simulink model "CubeSatModel_nopert"  (R2024a)
settings: Solver=FixedStepAuto  StartTime=0.0  StopTime=5467.6512  FixedStep=0.5  RelTol=1e-6  AbsTol=1e-7
PostLoadFcn:
  | if builtin('license','test','Virtual_Reality_Toolbox')
  |     set_param([bdroot(gcs) '/Simulink 3D Animation'], 'enableVis', 'on')
  | else
  |     set_param([bdroot(gcs) '/Simulink 3D Animation'], 'enableVis', 'off')
  | end
InitFcn:
  | if strcmp(get_param([bdroot(gcs) '/Simulink 3D Animation'], 'enableVis'), 'on')
  |     if ~builtin('license','checkout','Virtual_Reality_Toolbox')
  |         error(message('aeroblks_cubesat:cubesat:licenseFailAnimTemplate'));
  |     end
  | end
model workspace (MATLAB code in the model file + MAT data in the model file):
  aeroCoeff.Cl0 = 0.000591
  aeroCoeff.Cl_beta = -0.0618
  aeroCoeff.Cl_da = -0.09917
  aeroCoeff.Cl_da_alpha = -0.08269
  aeroCoeff.Cl_dr = 0.006934
  aeroCoeff.Cl_p = -0.5045
  aeroCoeff.Cl_r = 0.1695
  aeroCoeff.Cm0 = 0.09448
  aeroCoeff.Cm_alpha = -0.6028
  aeroCoeff.Cm_alpha2 = -2.14
  aeroCoeff.Cm_beta2 = 0.6921
  aeroCoeff.Cm_de = -1.921
  aeroCoeff.Cm_df = 0.4072
  aeroCoeff.Cm_q = -15.56
  aeroCoeff.Cm_r = -0.3118
  aeroCoeff.Cn0 = -0.003117
  aeroCoeff.Cn_beta = 0.006719
  aeroCoeff.Cn_beta3 = 0.1373
  aeroCoeff.Cn_da = -0.003872
  aeroCoeff.Cn_dr = -0.08265
  aeroCoeff.Cn_p = -0.1585
  aeroCoeff.Cn_q = 0.1595
  aeroCoeff.Cn_r = -0.1112
  aeroCoeff.Cx0 = -0.03554
  aeroCoeff.Cx_alpha = 0.00292
  aeroCoeff.Cx_alpha2 = 5.459
  aeroCoeff.Cx_alpha3 = -5.162
  aeroCoeff.Cx_df = -0.09447
  aeroCoeff.Cx_df_alpha = 1.106
  aeroCoeff.Cx_dr = 0.03412
  aeroCoeff.Cx_q = -0.6748
  aeroCoeff.Cy0 = -0.002226
  aeroCoeff.Cy_beta = -0.7678
  aeroCoeff.Cy_da = -0.02956
  aeroCoeff.Cy_dr = 0.1158
  aeroCoeff.Cy_dr_alpha = 0.5238
  aeroCoeff.Cy_p = -0.124
  aeroCoeff.Cy_r = 0.3666
  aeroCoeff.Cz0 = -0.05504
  aeroCoeff.Cz_alpha = -5.578
  aeroCoeff.Cz_alpha3 = 3.442
  aeroCoeff.Cz_de = -0.398
  aeroCoeff.Cz_de_beta = -15.93
  aeroCoeff.Cz_df = -1.377
  aeroCoeff.Cz_df_alpha = -1.261
  aeroCoeff.Cz_q = -2.988
  environment.EarthRefAlt = 0
  initCond.x0 = [0 0 -2202]
  initCond.v0 = [44.54 2.714 5.836]
  initCond.euler0 = [0 0.1308996939 0]
  initCond.w0 = [0 0 0]
  inputs0.time = 0
  inputs0.signals(1).dimensions = 1
  inputs0.signals(1).values = -0.104711430294
  inputs0.signals(2).dimensions = 1
  inputs0.signals(2).values = -0.0698725229544
  inputs0.signals(3).dimensions = 1
  inputs0.signals(3).values = -0.000215042330254
  states0.time = 0
  states0.signals(1).values = [0 0 -2202]
  states0.signals(1).dimensions = 3
  states0.signals(1).label = 'CSTATE'
  states0.signals(1).blockName = 'asb6DOFAirframeTemplate/6DOF EOM/6DOF (Euler Angles)/xe,ye,ze'
  states0.signals(1).stateName = ''
  states0.signals(1).inReferencedModel = 0
  states0.signals(1).sampleTime = [0 0]
  states0.signals(2).values = [0.128665353089 0.259337659946 -0.178947917154]
  states0.signals(2).dimensions = 3
  states0.signals(2).label = 'CSTATE'
  states0.signals(2).blockName = 'asb6DOFAirframeTemplate/6DOF EOM/6DOF (Euler Angles)/Calculate DCM &
    | Euler Angles/phi
    | theta
    | psi'
  states0.signals(2).stateName = ''
  states0.signals(2).inReferencedModel = 0
  states0.signals(2).sampleTime = [0 0]
  states0.signals(3).values = [36.9119692666 8.10720863264 8.82591882596]
  states0.signals(3).dimensions = 3
  states0.signals(3).label = 'CSTATE'
  states0.signals(3).blockName = 'asb6DOFAirframeTemplate/6DOF EOM/6DOF (Euler Angles)/ub,vb,wb'
  states0.signals(3).stateName = ''
  states0.signals(3).inReferencedModel = 0
  states0.signals(3).sampleTime = [0 0]
  states0.signals(4).values = [0 0 0]
  states0.signals(4).dimensions = 3
  states0.signals(4).label = 'CSTATE'
  states0.signals(4).blockName = 'asb6DOFAirframeTemplate/6DOF EOM/6DOF (Euler Angles)/p,q,r '
  states0.signals(4).stateName = ''
  states0.signals(4).inReferencedModel = 0
  states0.signals(4).sampleTime = [0 0]
  states0.signals(5).values = [0 0]
  states0.signals(5).dimensions = 2
  states0.signals(5).label = 'CSTATE'
  states0.signals(5).blockName = 'asb6DOFAirframeTemplate/Environment Model/Dryden Wind Turbulence Model 
    | (Continuous (+q +r))/Filters on velocities/Hwgw(s)/wg_p1'
  states0.signals(5).stateName = ''
  states0.signals(5).inReferencedModel = 0
  states0.signals(5).sampleTime = [0 0]
  states0.signals(6).values = [0 0]
  states0.signals(6).dimensions = 2
  states0.signals(6).label = 'CSTATE'
  states0.signals(6).blockName = 'asb6DOFAirframeTemplate/Environment Model/Dryden Wind Turbulence Model 
    | (Continuous (+q +r))/Filters on velocities/Hwgw(s)/wg_p2'
  states0.signals(6).stateName = ''
  states0.signals(6).inReferencedModel = 0
  states0.signals(6).sampleTime = [0 0]
  states0.signals(7).values = [0 0]
  states0.signals(7).dimensions = 2
  states0.signals(7).label = 'CSTATE'
  states0.signals(7).blockName = 'asb6DOFAirframeTemplate/Environment Model/Dryden Wind Turbulence Model 
    | (Continuous (+q +r))/Filters on velocities/Hvgw(s)/vg_p1'
  states0.signals(7).stateName = ''
  states0.signals(7).inReferencedModel = 0
  states0.signals(7).sampleTime = [0 0]
  states0.signals(8).values = [0 0]
  states0.signals(8).dimensions = 2
  states0.signals(8).label = 'CSTATE'
  states0.signals(8).blockName = 'asb6DOFAirframeTemplate/Environment Model/Dryden Wind Turbulence Model 
    | (Continuous (+q +r))/Filters on velocities/Hvgw(s)/vgw_p2'
  states0.signals(8).stateName = ''
  states0.signals(8).inReferencedModel = 0
  states0.signals(8).sampleTime = [0 0]
  states0.signals(9).values = [0 0]
  states0.signals(9).dimensions = 2
  states0.signals(9).label = 'CSTATE'
  states0.signals(9).blockName = 'asb6DOFAirframeTemplate/Environment Model/Dryden Wind Turbulence Model 
    | (Continuous (+q +r))/Filters on velocities/Hugw(s)/ug_p'
  states0.signals(9).stateName = ''
  states0.signals(9).inReferencedModel = 0
  states0.signals(9).sampleTime = [0 0]
  states0.signals(10).values = [0 0]
  states0.signals(10).dimensions = 2
  states0.signals(10).label = 'CSTATE'
  states0.signals(10).blockName = 'asb6DOFAirframeTemplate/Environment Model/Dryden Wind Turbulence Model 
    | (Continuous (+q +r))/Filters on angular rates/Hrgw/rgw_p'
  states0.signals(10).stateName = ''
  states0.signals(10).inReferencedModel = 0
  states0.signals(10).sampleTime = [0 0]
  states0.signals(11).values = [0 0]
  states0.signals(11).dimensions = 2
  states0.signals(11).label = 'CSTATE'
  states0.signals(11).blockName = 'asb6DOFAirframeTemplate/Environment Model/Dryden Wind Turbulence Model 
    | (Continuous (+q +r))/Filters on angular rates/Hqgw/qgw_p'
  states0.signals(11).stateName = ''
  states0.signals(11).inReferencedModel = 0
  states0.signals(11).sampleTime = [0 0]
  states0.signals(12).values = [0 0]
  states0.signals(12).dimensions = 2
  states0.signals(12).label = 'CSTATE'
  states0.signals(12).blockName = 'asb6DOFAirframeTemplate/Environment Model/Dryden Wind Turbulence Model 
    | (Continuous (+q +r))/Filters on angular rates/Hpgw/pgw_p'
  states0.signals(12).stateName = ''
  states0.signals(12).inReferencedModel = 0
  states0.signals(12).sampleTime = [0 0]
  vehicle.Sref = 23.23
  vehicle.cbar = 1.5875
  vehicle.bref = 14.63
  vehicle.CG = [0 0 0]
  vehicle.CP = [0 0 0]
  vehicle.inertia = [5788  0  117.6; 0  6928.9  0; -117.6  0  11578.3]
  vehicle.acMass = 2288.231
  vehicle.Thrust = 2300
  vehicle.aileron_max = 0.523598775598
  vehicle.aileron_min = -0.523598775598
  vehicle.elevator_max = 0.523598775598
  vehicle.elevator_min = -0.523598775598
  vehicle.rudder_max = 1.0471975512
  vehicle.rudder_min = -1.0471975512
  other statements: initialize6DOFSkyHogg;
libraries: aerolibutil x12, sharedutil x4, aerolibconvert2 x4, aerolibcubesatveh x1, aerolibobsolete x1, aerolibattitudesys x1, simulink x1, vrlib x1
settings Model: Creator=sandr  LastModifiedBy=sandr
settings SolverCC: AlgebraicLoopSolver=TrustRegion  AutoInsertRateTranBlk=on  InsertRTBMode=Never (minimum delay)  MinimalZcImpactIntegration=on  MaxZcPerStep=1
settings DataIOCC: SignalLogging=off  DSMLogging=off  SaveTime=off
settings OptimizationCC: EnhancedBackFolding=on  StrengthReduction=on  InitFltsAndDblsToZero=on  DifferentSizesBufferReuse=on
settings DebuggingCC: WriteAfterWriteMsg=DisableAll  AlgebraicLoopMsg=none  FcnCallInpInsideContextMsg=warning  UniqueDataStoreMsg=error  RootOutportRequireBusObject=none  StateNameClashWarn=warning  PregeneratedLibrarySubsystemCodeDiagnostic=none  StrictBusMsg=ErrorOnBusTreatedAsVector  SFUnexpectedBacktrackingDiag=warning  SFNoUnconditionalDefaultTransitionDiag=warning  SFExecutionAtInitializationDiag=none  ArithmeticOperatorsInVariantConditions=warning
settings ModelReferenceCC: EnableRefExpFcnMdlSchedulingChecks=on  PropagateSignalLabelsOutOfModel=off
settings SFSimCC: SimUseLocalCustomCode=off
settings RTWCC: RTWUseLocalCustomCode=off  GPUComputeCapability=3.5  DLArmComputeVersion=19.05
settings CodeAppCC: StateflowObjectComments=on

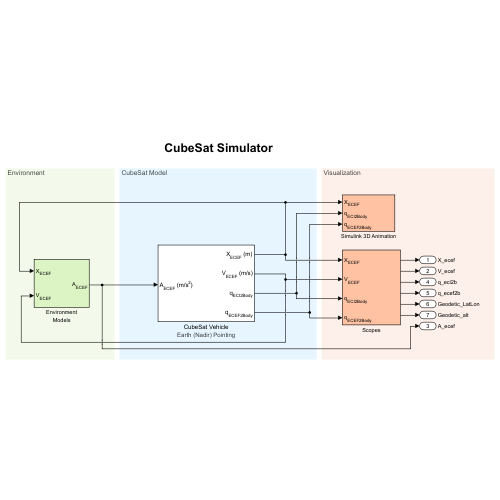
[thumbnail: Simulink's stored preview of the top-level diagram]
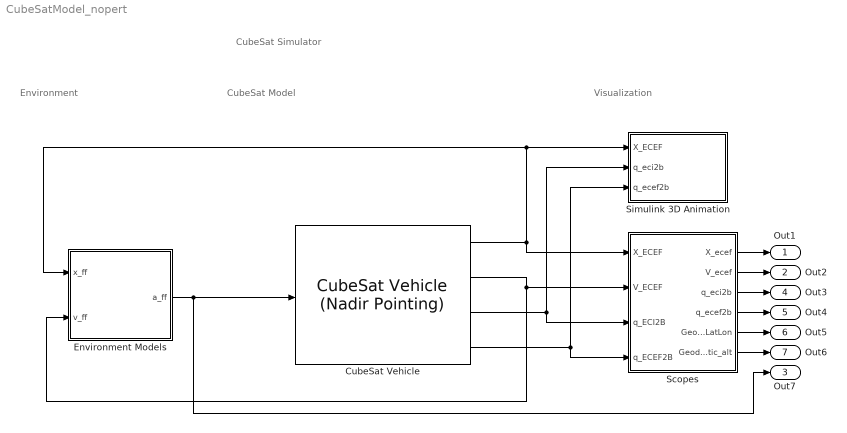
== system CubeSatModel_nopert ==
  note: CubeSat Simulator
  note: Visualization
  note: Environment
  note: CubeSat Model
  CubeSat Vehicle : aerolibcubesatveh/CubeSat Vehicle (Nadir Pointing)  sim_t0=2456824  method=Keplerian Orbital Elements  epoch=2456824  a=mission.CubeSat.SemiMajorAxis  ecc=mission.CubeSat.Eccentricity  incl=mission.CubeSat.Inclination  omega=mission.CubeSat.RAAN  argp=mission.CubeSat.ArgOfPeriapsis  nu=mission.CubeSat.TrueAnomaly  truelon=0  arglat=0  lonper=0  r_eci=[0 0 0]  v_eci=[0 0 0]  r_ecef=[0 0 0]  v_ecef=[0 0 0]  lla=[0 0 0]  v_ned=[0 0 0]  euler=mission.CubeSat.Euler  pqr=mission.CubeSat.AngularRate  pointingMode=Earth (Nadir) Pointing  firstAlignExt=Dialog  firstAlign=[0 0 1]  secondAlignExt=Dialog  secondAlign=[0 1 0]  constraintCoord=ECI Axes  firstRefExt=Dialog  firstRef=[1 0 0]  secondRefExt=Dialog  secondRef=[0 0 1]  missionRTSource=Dialog  missionRT=6*60*60  missionGS=[42, -71]  missionTOICheck=on  missionTOI=[]  missionEta=55
      settings: AttributesFormatString=%<pointingMode>
  Environment Models : Subsystem
      mask Display:
      | port_label('input', 1, 'X_{ECEF}','texmode','on')
      | port_label('input', 2, 'V_{ECEF}','texmode','on')
      | port_label('output', 1, 'A_{ECEF}','texmode','on')
  Scopes : Subsystem  VariantControl=visOff
      mask Display:
      | port_label('input', 1, 'X_{ECEF}','texmode','on')
      | port_label('input', 2, 'V_{ECEF}','texmode','on')
      | port_label('input', 3, 'q_{ECI2Body}','texmode','on')
      | port_label('input', 4, 'q_{ECEF2Body}','texmode','on')
  Simulink 3D Animation : Subsystem  mask(Set Animation Properties){enableVis=on, startDate=2458488, visSampleTime=5, cubesatSize=2e5, showAntenna=on, antennaHeight=1e6, antennaHalfAngle=25}
      mask prompts: enableVis "spacecraft:cubesat:AnimEnableVis"; startDate "spacecraft:cubesat:StartDate"; visSampleTime "spacecraft:cubesat:AnimSampleTime"; cubesatSize "spacecraft:cubesat:MdlSize"; showAntenna "spacecraft:cubesat:ShowCone"; antennaHeight "spacecraft:cubesat:ConeHeight"; antennaHalfAngle "spacecraft:cubesat:ConeAngle"
      mask help: spacecraft:cubesat:VisBlockDesc
      settings: OpenFcn=|
      | if ~builtin('license','test','virtual_reality_toolbox')
      |     set_param(gcb, 'enableVis', 'off');
      | end
      | open_system(gcb,'mask');
      mask Callback enableVis:
      | if strcmp(get_param(gcb,'enableVis'), 'on')
      |     [licAvail, ~] = builtin('license','checkout','Virtual_Reality_Toolbox');
      |     if licAvail
      |         enable = repmat({'on'},7,1);
      |         set_param(gcb, 'Commented', 'off');
      |     else
      |         enable = repmat({'off'},7,1);
      |         set_param(gcb, 'Commented', 'on');
      |         set_param(gcb,'enableVis', 'off');
      |     end
      |     clear licAvail
      | else
      |     enable = repmat({'off'},7,1);
      |     set_param(gcb, 'Commented', 'on');
      | end
      | enable{1} = 'on';
      | set_param(gcb,'MaskEnables', enable);
      | clear enable
      mask Callback showAntenna:
      | if strcmp(get_param(gcb, 'enableVis'), 'on')
      |     enable = get_param(gcb,'MaskEnables');
      |     if strcmp(get_param(gcb, 'showAntenna'), 'off')
      |         enable(6:7) = {'off'};
      |     else
      |         enable(6:7) = {'on'};
      |     end
      |     set_param(gcb,'MaskEnables', enable);
      |     clear enable
      | end
      mask DialogControl enableVis Prompt: Enable visualization with Simulink 3D Animation
      mask DialogControl vrOpenBtn Prompt: spacecraft:cubesat:AnimOpenBtn
      mask DialogControl vrOpenBtn Callback:
      | if builtin('license','checkout','Virtual_Reality_Toolbox')
      |     vrmfunc('FnOpen',getSimulinkBlockHandle([gcb '/VR Sink']));
      | end
      mask DialogControl startDate Prompt: Start date [Julian date]:
      mask DialogControl startDate Tooltip: spacecraft:cubesat:StartDateTT
      mask DialogControl visSampleTime Prompt: Animation refresh rate:
      mask DialogControl visSampleTime Tooltip: spacecraft:cubesat:AnimSampleTimeTT
      mask DialogControl cubesatSize Prompt: CubeSat display size [m]:
      mask DialogControl cubesatSize Tooltip: spacecraft:cubesat:MdlSizeTT
      mask DialogControl Container3 Prompt: spacecraft:cubesat:AntennaPropArea
      mask DialogControl showAntenna Prompt: Show antenna cone in animation
      mask DialogControl showAntenna Tooltip: spacecraft:cubesat:ShowConeTT
      mask DialogControl antennaHeight Prompt: Antenna cone height [m]:
      mask DialogControl antennaHeight Tooltip: spacecraft:cubesat:ConeHeightTT
      mask DialogControl antennaHalfAngle Prompt: Antenna cone half angle [deg]:
      mask DialogControl antennaHalfAngle Tooltip: spacecraft:cubesat:ConeAngleTT
      mask Display:
      | port_label('input', 1, 'X_{ECEF}','texmode','on')
      | port_label('input', 2, 'q_{ECI2Body}','texmode','on')
      | port_label('input', 3, 'q_{ECEF2Body}','texmode','on')
  Out1 : Outport  SignalName=X_ecef
  Out2 : Outport  Port=2  SignalName=V_ecef
  Out7 : Outport  Port=3  SignalName=A_ecef
  Out3 : Outport  Port=4  SignalName=q_eci2b
  Out4 : Outport  Port=5  SignalName=q_ecef2b
  Out5 : Outport  Port=6  SignalName=Geodetic_LatLon
  Out6 : Outport  Port=7  SignalName=Geodetic_alt
  wires:
  Environment Models/1(a_ff) -> Out7/1, CubeSat Vehicle/1
  CubeSat Vehicle/1 -> Scopes/1(X_ECEF), Environment Models/1(x_ff), Simulink 3D Animation/1(X_ECEF)
  CubeSat Vehicle/3 -> Simulink 3D Animation/2(q_eci2b), Scopes/3(q_ECI2B)
  CubeSat Vehicle/2 -> Environment Models/2(v_ff), Scopes/2(V_ECEF)
  CubeSat Vehicle/4 -> Simulink 3D Animation/3(q_ecef2b), Scopes/4(q_ECEF2B)
  Scopes/1(X_ecef) -> Out1/1
  Scopes/2(V_ecef) -> Out2/1
  Scopes/3(q_eci2b) -> Out3/1
  Scopes/4(q_ecef2b) -> Out4/1
  Scopes/5(Geodetic_LatLon) -> Out5/1
  Scopes/6(Geodetic_alt) -> Out6/1

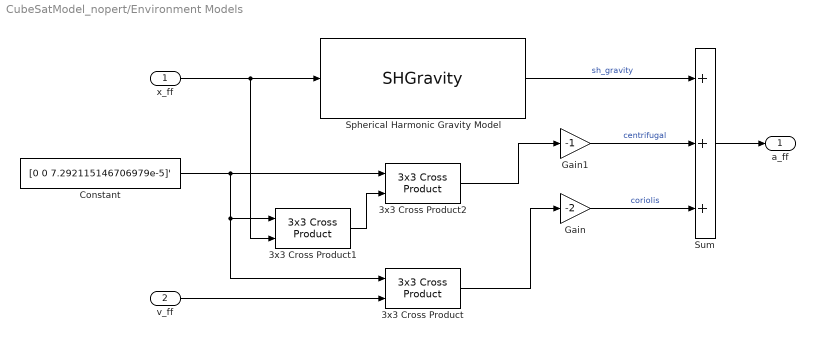
== system CubeSatModel_nopert/Environment Models ==
  x_ff : Inport  Unit=m  PortDimensions=3
  v_ff : Inport  Port=2  Unit=m/s  PortDimensions=3
  3x3 Cross Product : sharedutil/3x3 Cross Product  aMode=aMode
  3x3 Cross Product1 : sharedutil/3x3 Cross Product  aMode=aMode
  3x3 Cross Product2 : sharedutil/3x3 Cross Product  aMode=aMode
  Constant : Constant  Value=[0 0 7.292115146706979e-5]'
  Gain : Gain  Gain=-2
  Gain1 : Gain  Gain=-1
  Spherical Harmonic Gravity Model : SHGravity  degree=40
  Sum : Sum  Inputs=+++
  a_ff : Outport  Unit=m/s^2  PortDimensions=3
  wires:
  Gain/1 -> Sum/3  "coriolis"
  v_ff/1 -> 3x3 Cross Product/2
  x_ff/1 -> Spherical Harmonic Gravity Model/1, 3x3 Cross Product1/2
  Sum/1 -> a_ff/1
  3x3 Cross Product2/1 -> Gain1/1
  Gain1/1 -> Sum/2  "centrifugal"
  Spherical Harmonic Gravity Model/1 -> Sum/1  "sh_gravity"
  3x3 Cross Product1/1 -> 3x3 Cross Product2/2
  Constant/1 -> 3x3 Cross Product2/1, 3x3 Cross Product/1, 3x3 Cross Product1/1
  3x3 Cross Product/1 -> Gain/1

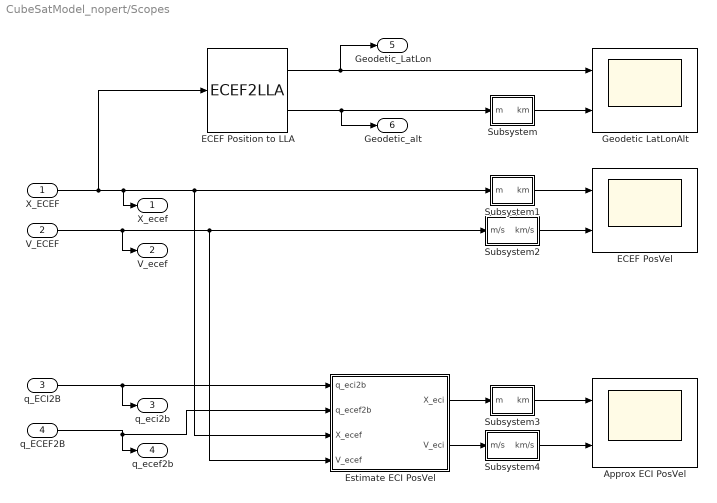
== system CubeSatModel_nopert/Scopes ==
  X_ECEF : Inport
  V_ECEF : Inport  Port=2
  q_ECI2B : Inport  Port=3
  q_ECEF2B : Inport  Port=4
  Approx ECI PosVel : Scope  NumInputPorts=2
  ECEF PosVel : Scope  NumInputPorts=2
  ECEF Position to LLA : ECEF2LLA  R=6378137
  Estimate ECI PosVel : Subsystem
  Geodetic LatLonAlt : Scope  NumInputPorts=2
  Subsystem : Subsystem
  Subsystem1 : Subsystem
  Subsystem2 : Subsystem
  Subsystem3 : Subsystem
  Subsystem4 : Subsystem
  X_ecef : Outport
  V_ecef : Outport  Port=2
  q_eci2b : Outport  Port=3
  q_ecef2b : Outport  Port=4
  Geodetic_LatLon : Outport  Port=5
  Geodetic_alt : Outport  Port=6
  wires:
  V_ECEF/1 -> V_ecef/1, Subsystem2/1(m/s), Estimate ECI PosVel/4(V_ecef)
  X_ECEF/1 -> X_ecef/1, Subsystem1/1(m), Estimate ECI PosVel/3(X_ecef), ECEF Position to LLA/1
  q_ECI2B/1 -> q_eci2b/1, Estimate ECI PosVel/1(q_eci2b)
  Estimate ECI PosVel/2(V_eci) -> Subsystem4/1(m/s)
  Estimate ECI PosVel/1(X_eci) -> Subsystem3/1(m)
  ECEF Position to LLA/2 -> Geodetic_alt/1, Subsystem/1(m)
  Subsystem/1(km) -> Geodetic LatLonAlt/2
  Subsystem1/1(km) -> ECEF PosVel/1
  Subsystem2/1(km/s) -> ECEF PosVel/2
  Subsystem3/1(km) -> Approx ECI PosVel/1
  Subsystem4/1(km/s) -> Approx ECI PosVel/2
  ECEF Position to LLA/1 -> Geodetic LatLonAlt/1, Geodetic_LatLon/1
  q_ECEF2B/1 -> q_ecef2b/1, Estimate ECI PosVel/2(q_ecef2b)

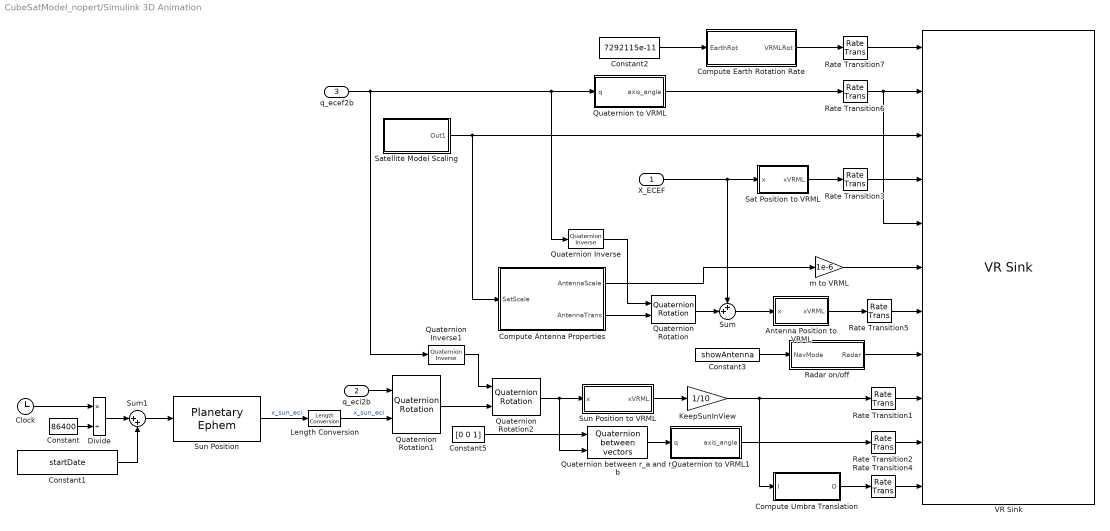
== system CubeSatModel_nopert/Simulink 3D Animation ==
  X_ECEF : Inport
  q_eci2b : Inport  Port=2
  q_ecef2b : Inport  Port=3
  Antenna Position to VRML : Subsystem
  Clock : Clock
  Compute Antenna Properties : Subsystem
  Compute Earth Rotation Rate : Subsystem
  Compute Umbra Translation : Subsystem
  Constant : Constant  Value=86400
  Constant1 : Constant  RequirementInfo={} %GIDa_d3dce1ea_7a4c_4489_9b49_860fce94c68a  Value=startDate  SampleTime=visSampleTime
  Constant2 : Constant  RequirementInfo={} %GIDa_a027479b_4c7b_4f1d_b86b_1fc869131b24  Value=7292115e-11
  Constant3 : Constant  Value=showAntenna
  Constant5 : Constant  Value=[0 0 1]
  Divide : Product  Inputs=*/
  KeepSunInView : Gain  Gain=1/10
  Length Conversion : aerolibconvert2/Length Conversion  IU=km  OU=m
  Quaternion Inverse : aerolibutil/Quaternion Inverse
  Quaternion Inverse1 : aerolibutil/Quaternion Inverse
  Quaternion Rotation : aerolibutil/Quaternion Rotation
  Quaternion Rotation1 : aerolibutil/Quaternion Rotation
  Quaternion Rotation2 : aerolibutil/Quaternion Rotation
  Quaternion between r_a and r_b : aerolibattitudesys/Quaternion between vectors
  Quaternion to VRML : Subsystem
  Quaternion to VRML1 : Subsystem
  Radar on/off : Subsystem
  Rate Transition{1..7} (7 alike) : RateTransition
  Sat Position to VRML : Subsystem
  Satellite Model Scaling : Subsystem
  Sum : Sum  Inputs=++|
  Sum1 : Sum  Inputs=|++
  Sun Position : PlanetaryEphem  ephemerisModel=DE421  target=Sun  outputVelocity=off
  Sun Position to VRML : Subsystem
  VR Sink : vrlib/VR Sink  InstantiateOnLoad=on  SampleTime=visSampleTime  ViewEnable=on  RemoteChange=off  RemoteView=off  FieldsWritten=Earth.rotation.4.1.1.double#Satellite.rotation.4.1.1.double#Satellite.scale.3.1.1.double#Satellite.translation.3.1.1.double#AntennaCone.rotation.4.1.1.double#AntennaCone.scale.3.1.1.double#AntennaCone.translation.3.1.1.double#AntennaMaterial.transparency.1.1.1.double#Sun.translation.3.1.1.double#Umbra.rotation.4.1.1.double#Umbra.translation.3.1.1.double  WorldFileName=cubesatAnim.wrl  WorldDescription=CubeSat Orbit Animation  AutoView=on  VideoDimensions=[]  AllowVariableSize=off
  m to VRML : Gain  Gain=1e-6
  wires:
  Quaternion to VRML1/1(axis_angle) -> Rate Transition2/1
  Quaternion between r_a and r_b/1 -> Quaternion to VRML1/1(q)
  Constant2/1 -> Compute Earth Rotation Rate/1(EarthRot)
  Compute Antenna Properties/1(AntennaScale) -> m to VRML/1
  Quaternion to VRML/1(axis_angle) -> Rate Transition6/1
  Compute Umbra Translation/1(O) -> Rate Transition4/1
  q_eci2b/1 -> Quaternion Rotation1/1
  Quaternion Rotation2/1 -> Sun Position to VRML/1(x), Quaternion between r_a and r_b/2
  Constant5/1 -> Quaternion between r_a and r_b/1
  KeepSunInView/1 -> Compute Umbra Translation/1(I), Rate Transition1/1
  Sun Position to VRML/1(xVRML) -> KeepSunInView/1
  Sat Position to VRML/1(xVRML) -> Rate Transition3/1
  Compute Antenna Properties/2(AntennaTrans) -> Quaternion Rotation/2
  Satellite Model Scaling/1(Out1) -> VR Sink/3, Compute Antenna Properties/1(SatScale)
  Constant3/1 -> Radar on/off/1(NavMode)
  q_ecef2b/1 -> Quaternion Inverse/1, Quaternion to VRML/1(q), Quaternion Inverse1/1
  Quaternion Rotation1/1 -> Quaternion Rotation2/2
  Compute Earth Rotation Rate/1(VRMLRot) -> Rate Transition7/1
  Antenna Position to VRML/1(xVRML) -> Rate Transition5/1
  Quaternion Inverse/1 -> Quaternion Rotation/1
  X_ECEF/1 -> Sat Position to VRML/1(x), Sum/1
  Quaternion Rotation/1 -> Sum/2
  Sum/1 -> Antenna Position to VRML/1(x)
  Quaternion Inverse1/1 -> Quaternion Rotation2/1
  Rate Transition4/1 -> VR Sink/11
  Rate Transition2/1 -> VR Sink/10
  Rate Transition1/1 -> VR Sink/9
  Rate Transition5/1 -> VR Sink/7
  m to VRML/1 -> VR Sink/6
  Rate Transition3/1 -> VR Sink/4
  Rate Transition7/1 -> VR Sink/1
  Rate Transition6/1 -> VR Sink/5, VR Sink/2
  Constant1/1 -> Sum1/2
  Divide/1 -> Sum1/1
  Constant/1 -> Divide/2
  Sun Position/1 -> Length Conversion/1  "x_sun_eci"
  Clock/1 -> Divide/1
  Length Conversion/1 -> Quaternion Rotation1/2  "x_sun_eci"
  Sum1/1 -> Sun Position/1
  Radar on/off/1(Radar) -> VR Sink/8

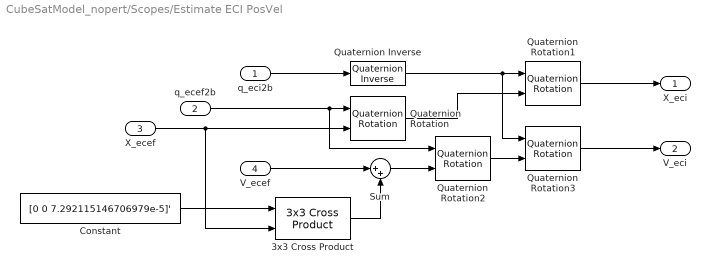
== system CubeSatModel_nopert/Scopes/Estimate ECI PosVel ==
  q_eci2b : Inport
  q_ecef2b : Inport  Port=2
  X_ecef : Inport  Port=3
  V_ecef : Inport  Port=4
  3x3 Cross Product : sharedutil/3x3 Cross Product  aMode=aMode
  Constant : Constant  Value=[0 0 7.292115146706979e-5]'
  Quaternion Inverse : aerolibutil/Quaternion Inverse
  Quaternion Rotation{,1..3} (4 alike) : aerolibutil/Quaternion Rotation
  Sum : Sum  Inputs=|++
  X_eci : Outport  VectorParamsAs1DForOutWhenUnconnected=off
  V_eci : Outport  Port=2  VectorParamsAs1DForOutWhenUnconnected=off
  wires:
  Quaternion Rotation3/1 -> V_eci/1
  X_ecef/1 -> Quaternion Rotation/2, 3x3 Cross Product/2
  Quaternion Rotation1/1 -> X_eci/1
  q_eci2b/1 -> Quaternion Inverse/1
  Quaternion Rotation2/1 -> Quaternion Rotation3/2
  Constant/1 -> 3x3 Cross Product/1
  Quaternion Inverse/1 -> Quaternion Rotation1/1, Quaternion Rotation3/1
  q_ecef2b/1 -> Quaternion Rotation2/1, Quaternion Rotation/1
  Quaternion Rotation/1 -> Quaternion Rotation1/2
  V_ecef/1 -> Sum/1
  3x3 Cross Product/1 -> Sum/2
  Sum/1 -> Quaternion Rotation2/2

== system CubeSatModel_nopert/Scopes/Subsystem ==
  m : Inport  Unit=m
  Unit Conversion : UnitConversion
  km : Outport  Unit=km  VectorParamsAs1DForOutWhenUnconnected=off
  wires:
  Unit Conversion/1 -> km/1
  m/1 -> Unit Conversion/1

== system CubeSatModel_nopert/Scopes/Subsystem1 ==
  m : Inport  Unit=m
  Unit Conversion : UnitConversion
  km : Outport  Unit=km  VectorParamsAs1DForOutWhenUnconnected=off
  wires:
  m/1 -> Unit Conversion/1
  Unit Conversion/1 -> km/1

== system CubeSatModel_nopert/Scopes/Subsystem2 ==
  m/s : Inport  Unit=m/s
  Unit Conversion : UnitConversion
  km/s : Outport  Unit=km/s  VectorParamsAs1DForOutWhenUnconnected=off
  wires:
  Unit Conversion/1 -> km/s/1
  m/s/1 -> Unit Conversion/1

== system CubeSatModel_nopert/Scopes/Subsystem3 ==
  m : Inport  Unit=m
  Unit Conversion : UnitConversion
  km : Outport  Unit=km  VectorParamsAs1DForOutWhenUnconnected=off
  wires:
  m/1 -> Unit Conversion/1
  Unit Conversion/1 -> km/1

== system CubeSatModel_nopert/Scopes/Subsystem4 ==
  m/s : Inport  Unit=m/s
  Unit Conversion : UnitConversion
  km/s : Outport  Unit=km/s  VectorParamsAs1DForOutWhenUnconnected=off
  wires:
  Unit Conversion/1 -> km/s/1
  m/s/1 -> Unit Conversion/1

== system CubeSatModel_nopert/Simulink 3D Animation/Antenna Position to VRML ==
  x : Inport
  ECEF to VRML : Subsystem
  Length Conversion : aerolibconvert2/Length Conversion  IU=m  OU=km
  km to VRML units : Gain  Gain=1/1000
  xVRML : Outport  VectorParamsAs1DForOutWhenUnconnected=off
  wires:
  Length Conversion/1 -> km to VRML units/1
  km to VRML units/1 -> ECEF to VRML/1(M)
  x/1 -> Length Conversion/1
  ECEF to VRML/1(VR) -> xVRML/1

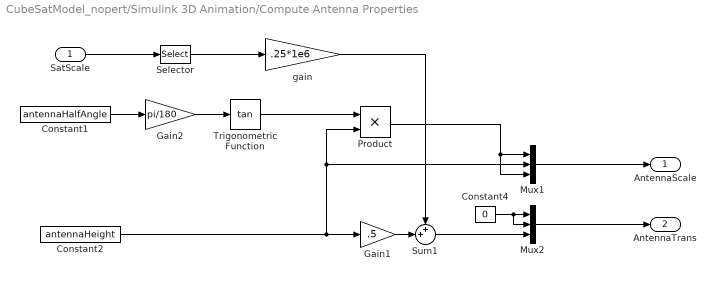
== system CubeSatModel_nopert/Simulink 3D Animation/Compute Antenna Properties ==
  SatScale : Inport
  Constant1 : Constant  Value=antennaHalfAngle
  Constant2 : Constant  Value=antennaHeight
  Constant4 : Constant  Value=0
  Gain1 : Gain  Gain=.5
  Gain2 : Gain  Gain=pi/180
  Mux1 : Mux  Inputs=3
  Mux2 : Mux  Inputs=3
  Product : Product
  Selector : Selector  InputPortWidth=3  IndexOptions=Index vector (dialog)  Indices=1  OutputSizes=1
  Sum1 : Sum  Inputs=++|
  Trigonometric Function : Trigonometry  Operator=tan
  gain : Gain  Gain=.25*1e6
  AntennaScale : Outport  VectorParamsAs1DForOutWhenUnconnected=off
  AntennaTrans : Outport  Port=2  VectorParamsAs1DForOutWhenUnconnected=off
  wires:
  Gain2/1 -> Trigonometric Function/1
  Constant4/1 -> Mux2/1, Mux2/2
  Sum1/1 -> Mux2/3
  Constant2/1 -> Gain1/1, Mux1/2, Product/2
  gain/1 -> Sum1/1
  Constant1/1 -> Gain2/1
  Product/1 -> Mux1/3, Mux1/1
  Gain1/1 -> Sum1/2
  Trigonometric Function/1 -> Product/1
  Mux2/1 -> AntennaTrans/1
  Mux1/1 -> AntennaScale/1
  SatScale/1 -> Selector/1
  Selector/1 -> gain/1

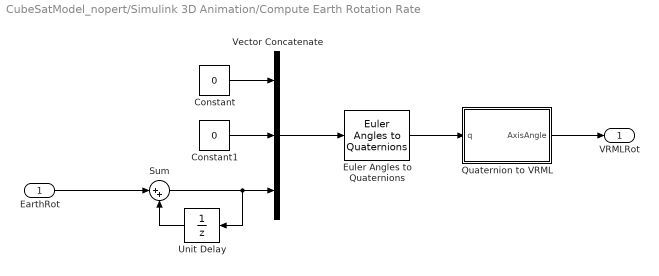
== system CubeSatModel_nopert/Simulink 3D Animation/Compute Earth Rotation Rate ==
  EarthRot : Inport
  Constant : Constant  Value=0
  Constant1 : Constant  Value=0
  Euler Angles to Quaternions : aerolibobsolete/Euler Angles to Quaternions
  Quaternion to VRML : Subsystem
  Sum : Sum  Inputs=|++
  Unit Delay : UnitDelay  SampleTime=-1  HasFrameUpgradeWarning=on
  Vector Concatenate : Concatenate  NumInputs=3
  VRMLRot : Outport  VectorParamsAs1DForOutWhenUnconnected=off
  wires:
  Quaternion to VRML/1(AxisAngle) -> VRMLRot/1
  Euler Angles to Quaternions/1 -> Quaternion to VRML/1(q)
  Vector Concatenate/1 -> Euler Angles to Quaternions/1
  Constant1/1 -> Vector Concatenate/2
  Constant/1 -> Vector Concatenate/1
  Sum/1 -> Unit Delay/1, Vector Concatenate/3
  Unit Delay/1 -> Sum/2
  EarthRot/1 -> Sum/1

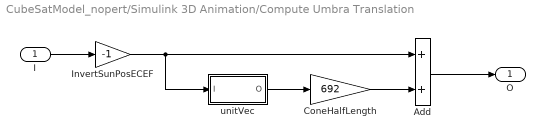
== system CubeSatModel_nopert/Simulink 3D Animation/Compute Umbra Translation ==
  I : Inport
  Add : Sum
  ConeHalfLength : Gain  Gain=692
  InvertSunPosECEF : Gain  Gain=-1
  unitVec : Subsystem
  O : Outport  VectorParamsAs1DForOutWhenUnconnected=off
  wires:
  ConeHalfLength/1 -> Add/2
  I/1 -> InvertSunPosECEF/1
  Add/1 -> O/1
  InvertSunPosECEF/1 -> unitVec/1(I), Add/1
  unitVec/1(O) -> ConeHalfLength/1

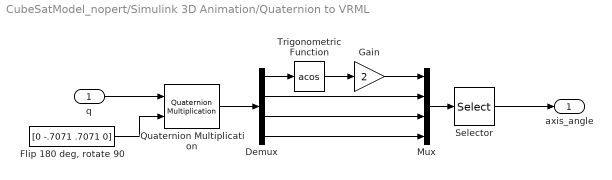
== system CubeSatModel_nopert/Simulink 3D Animation/Quaternion to VRML ==
  q : Inport
  Demux : Demux
  "Flip 180 deg, rotate 90" : Constant  Value=[0 -.7071 .7071 0]
  Gain : Gain  Gain=2
  Mux : Mux
  Quaternion Multiplication : aerolibutil/Quaternion Multiplication
  Selector : Selector  InputPortWidth=4  IndexOptions=Index vector (dialog)  Indices=[3 4 2 1]  OutputSizes=1
  Trigonometric Function : Trigonometry  Operator=acos
  axis_angle : Outport  VectorParamsAs1DForOutWhenUnconnected=off
  wires:
  Demux/4 -> Mux/4
  Demux/3 -> Mux/3
  Demux/2 -> Mux/2
  Gain/1 -> Mux/1
  Selector/1 -> axis_angle/1
  q/1 -> Quaternion Multiplication/1
  Mux/1 -> Selector/1
  Trigonometric Function/1 -> Gain/1
  Demux/1 -> Trigonometric Function/1
  "Flip 180 deg, rotate 90"/1 -> Quaternion Multiplication/2
  Quaternion Multiplication/1 -> Demux/1

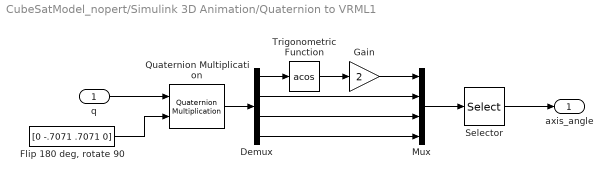
== system CubeSatModel_nopert/Simulink 3D Animation/Quaternion to VRML1 ==
  q : Inport
  Demux : Demux
  "Flip 180 deg, rotate 90" : Constant  Value=[0 -.7071 .7071 0]
  Gain : Gain  Gain=2
  Mux : Mux
  Quaternion Multiplication : aerolibutil/Quaternion Multiplication
  Selector : Selector  InputPortWidth=4  IndexOptions=Index vector (dialog)  Indices=[3 4 2 1]  OutputSizes=1
  Trigonometric Function : Trigonometry  Operator=acos
  axis_angle : Outport  VectorParamsAs1DForOutWhenUnconnected=off
  wires:
  Demux/4 -> Mux/4
  Demux/3 -> Mux/3
  Demux/2 -> Mux/2
  Gain/1 -> Mux/1
  Selector/1 -> axis_angle/1
  Mux/1 -> Selector/1
  Trigonometric Function/1 -> Gain/1
  Demux/1 -> Trigonometric Function/1
  "Flip 180 deg, rotate 90"/1 -> Quaternion Multiplication/2
  q/1 -> Quaternion Multiplication/1
  Quaternion Multiplication/1 -> Demux/1

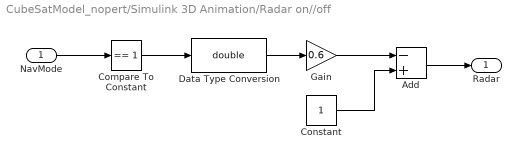
== system CubeSatModel_nopert/Simulink 3D Animation/Radar on//off ==
  NavMode : Inport
  Add : Sum  Inputs=-+
  Compare To Constant : simulink/Logic and Bit Operations/Compare To Constant  relop===  const=1  OutDataTypeStr=boolean  ZeroCross=off
  Constant : Constant
  Data Type Conversion : DataTypeConversion  OutDataTypeStr=double  SaturateOnIntegerOverflow=off  RndMeth=Floor
  Gain : Gain  Gain=0.6
  Radar : Outport  VectorParamsAs1DForOutWhenUnconnected=off
  wires:
  NavMode/1 -> Compare To Constant/1
  Compare To Constant/1 -> Data Type Conversion/1
  Data Type Conversion/1 -> Gain/1
  Gain/1 -> Add/1
  Constant/1 -> Add/2
  Add/1 -> Radar/1

== system CubeSatModel_nopert/Simulink 3D Animation/Sat Position to VRML ==
  x : Inport
  ECEF to VRML : Subsystem
  Length Conversion : aerolibconvert2/Length Conversion  IU=m  OU=km
  km to VRML units : Gain  Gain=1/1000
  xVRML : Outport  VectorParamsAs1DForOutWhenUnconnected=off
  wires:
  ECEF to VRML/1(VR) -> xVRML/1
  x/1 -> Length Conversion/1
  km to VRML units/1 -> ECEF to VRML/1(M)
  Length Conversion/1 -> km to VRML units/1

== system CubeSatModel_nopert/Simulink 3D Animation/Satellite Model Scaling ==
  Constant : Constant  Value=cubesatSize
  Mux : Mux  Inputs=3
  ScaleModelToVRML : Gain  Gain=1/.3e6
  Out1 : Outport  VectorParamsAs1DForOutWhenUnconnected=off
  wires:
  ScaleModelToVRML/1 -> Mux/3, Mux/1, Mux/2
  Constant/1 -> ScaleModelToVRML/1
  Mux/1 -> Out1/1

== system CubeSatModel_nopert/Simulink 3D Animation/Sun Position to VRML ==
  x : Inport
  ECEF to VRML : Subsystem
  Length Conversion : aerolibconvert2/Length Conversion  IU=m  OU=km
  km to VRML units : Gain  Gain=1/1000
  xVRML : Outport  VectorParamsAs1DForOutWhenUnconnected=off
  wires:
  ECEF to VRML/1(VR) -> xVRML/1
  x/1 -> Length Conversion/1
  km to VRML units/1 -> ECEF to VRML/1(M)
  Length Conversion/1 -> km to VRML units/1

== system CubeSatModel_nopert/Simulink 3D Animation/Antenna Position to VRML/ECEF to VRML ==
  M : Inport  PortDimensions=3
  Selector : Selector  InputPortWidth=3  IndexOptions=Index vector (dialog)  Indices=[2 3 1]  OutputSizes=1
  VR : Outport  PortDimensions=3  VectorParamsAs1DForOutWhenUnconnected=off
  wires:
  M/1 -> Selector/1
  Selector/1 -> VR/1

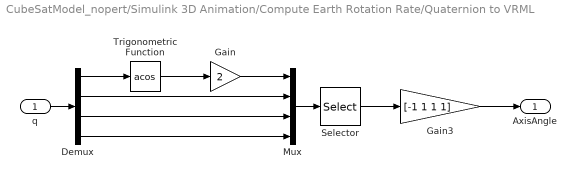
== system CubeSatModel_nopert/Simulink 3D Animation/Compute Earth Rotation Rate/Quaternion to VRML ==
  q : Inport
  Demux : Demux
  Gain : Gain  Gain=2
  Gain3 : Gain  Gain=[-1 1 1 1]
  Mux : Mux
  Selector : Selector  InputPortWidth=4  IndexOptions=Index vector (dialog)  Indices=[2 4 3 1]  OutputSizes=1
  Trigonometric Function : Trigonometry  Operator=acos
  AxisAngle : Outport  VectorParamsAs1DForOutWhenUnconnected=off
  wires:
  Demux/1 -> Trigonometric Function/1
  Trigonometric Function/1 -> Gain/1
  Mux/1 -> Selector/1
  q/1 -> Demux/1
  Gain3/1 -> AxisAngle/1
  Selector/1 -> Gain3/1
  Gain/1 -> Mux/1
  Demux/2 -> Mux/2
  Demux/3 -> Mux/3
  Demux/4 -> Mux/4

== system CubeSatModel_nopert/Simulink 3D Animation/Compute Umbra Translation/unitVec ==
  I : Inport
  Divide : Product  Inputs=*/
  Dot Product : DotProduct  OutDataTypeStr=Inherit: Inherit via internal rule
  Sqrt : Sqrt
  O : Outport  VectorParamsAs1DForOutWhenUnconnected=off
  wires:
  Dot Product/1 -> Sqrt/1
  I/1 -> Divide/1, Dot Product/1, Dot Product/2
  Divide/1 -> O/1
  Sqrt/1 -> Divide/2

== system CubeSatModel_nopert/Simulink 3D Animation/Sat Position to VRML/ECEF to VRML ==
  M : Inport  PortDimensions=3
  Selector : Selector  InputPortWidth=3  IndexOptions=Index vector (dialog)  Indices=[2 3 1]  OutputSizes=1
  VR : Outport  PortDimensions=3  VectorParamsAs1DForOutWhenUnconnected=off
  wires:
  M/1 -> Selector/1
  Selector/1 -> VR/1

== system CubeSatModel_nopert/Simulink 3D Animation/Sun Position to VRML/ECEF to VRML ==
  M : Inport  PortDimensions=3
  Selector : Selector  InputPortWidth=3  IndexOptions=Index vector (dialog)  Indices=[2 3 1]  OutputSizes=1
  VR : Outport  PortDimensions=3  VectorParamsAs1DForOutWhenUnconnected=off
  wires:
  M/1 -> Selector/1
  Selector/1 -> VR/1
